simulink model "es2_Q2_task1"  (R2022b)
settings: Solver=VariableStepAuto  StartTime=0.0  StopTime=100.0  RelTol=1e-3  AbsTol=1e-3  EnableMultiTasking=on
undefined symbols (not defined in the file): X, Y, Z
libraries: nesl_utility x37, sm_lib x25
settings Model: Creator=matteo  LastModifiedBy=veronicagavagna
settings SolverCC: AutoScaleAbsTol=off  AlgebraicLoopSolver=TrustRegion  MaxZcPerStep=1
settings DataIOCC: LimitDataPoints=on  MaxDataPoints=10000
settings OptimizationCC: LifeSpan=inf
settings DebuggingCC: UnconnectedInputMsg=warning  UnconnectedOutputMsg=warning  UnconnectedLineMsg=warning  AllowSymbolicDim=off  SFUnexpectedBacktrackingDiag=warning  SFNoUnconditionalDefaultTransitionDiag=warning  SFExecutionAtInitializationDiag=none  ArithmeticOperatorsInVariantConditions=warning
settings ModelReferenceCC: EnableRefExpFcnMdlSchedulingChecks=on
settings SFSimCC: SimUseLocalCustomCode=off  CustomCodeUndefinedFunction=UseInterfaceOnly
settings RTWCC: RTWUseLocalCustomCode=off  DLArmComputeVersion=19.05
settings CodeAppCC: StateflowObjectComments=on
settings GRTTargetCC: TargetLangStandard=C89/C90 (ANSI)
settings ConfigComp: CovMetricSettings=dw  CovSaveCumulativeToWorkspaceVar=on  CovSaveSingleToWorkspaceVar=on  CovExternalEMLEnable=off  CovSFcnEnable=off
settings SimscapeCC: SimscapeLogType=all  SimscapeLogSimulationStatistics=on  SimscapeLogDataHistory=10000

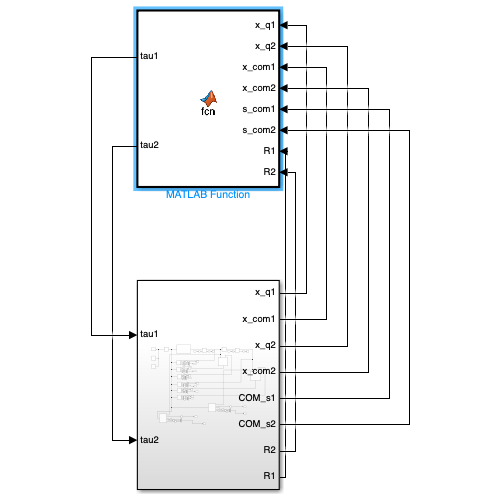
[thumbnail: Simulink's stored preview of the top-level diagram]
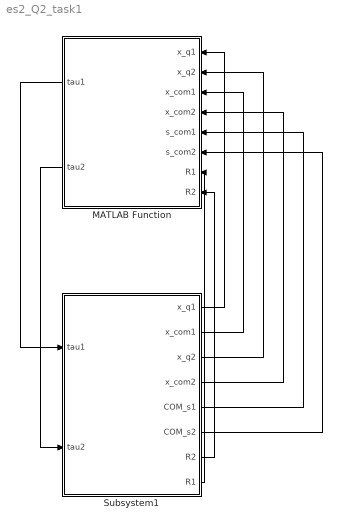
== system es2_Q2_task1 ==
  MATLAB Function : MATLAB Function  TreatAsAtomicUnit=on
  Subsystem1 : Subsystem
  wires:
  Subsystem1/1(x_q1) -> MATLAB Function/1(x_q1)
  Subsystem1/2(x_com1) -> MATLAB Function/3(x_com1)
  Subsystem1/3(x_q2) -> MATLAB Function/2(x_q2)
  Subsystem1/4(x_com2) -> MATLAB Function/4(x_com2)
  MATLAB Function/1(tau1) -> Subsystem1/1(tau1)
  MATLAB Function/2(tau2) -> Subsystem1/2(tau2)
  Subsystem1/5(COM_s1) -> MATLAB Function/5(s_com1)
  Subsystem1/6(COM_s2) -> MATLAB Function/6(s_com2)
  Subsystem1/7(R2) -> MATLAB Function/8(R2)
  Subsystem1/8(R1) -> MATLAB Function/7(R1)

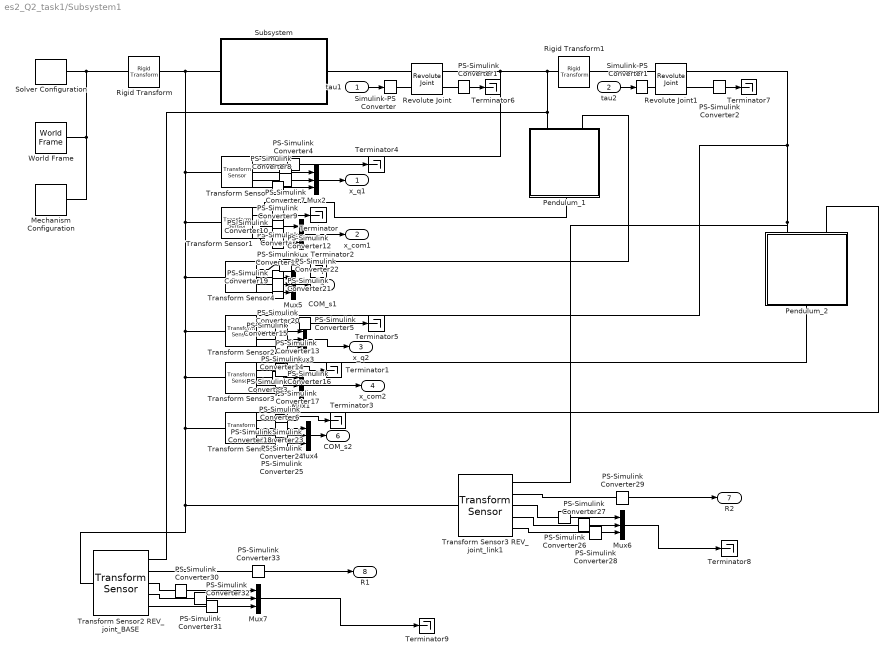
== system es2_Q2_task1/Subsystem1 ==
  tau1 : Inport
  tau2 : Inport  Port=2
  Mechanism Configuration : sm_lib/Utilities/Mechanism Configuration  UniformGravity=Constant  GravityVector=[0 0 -9.81]  GravityUnits=m/s^2  LinearizationDelta=0.001  JointModeTransitionNonlinearIterations=2
  Mux{,1..7} (8 alike) : Mux  Inputs=3
  PS-Simulink Converter{,1..33} (34 alike) : nesl_utility/PS-Simulink Converter  PhysicalDomain=network_engine_domain  SubClassName=ps_output  LeftPortType=input  RightPortType=output  PseudoPeriodic=off  Frequencies=[]  VectorFormat=inherit  Unit=inherit  AffineConversion=off
  Pendulum_1 : Subsystem
  Pendulum_2 : Subsystem
  Revolute Joint : sm_lib/Joints/Revolute Joint  JointMode=Normal  SenseConstraintForce=off  SenseConstraintForceX=off  SenseConstraintForceY=off  SenseConstraintForceZ=off  SenseConstraintTorque=off  SenseConstraintTorqueX=off  SenseConstraintTorqueY=off  SenseConstraintTorqueZ=off  SenseTotalForce=off  SenseTotalForceX=off  SenseTotalForceY=off  SenseTotalForceZ=off  SenseTotalTorque=off  SenseTotalTorqueX=off  SenseTotalTorqueY=off  SenseTotalTorqueZ=off  CompositeWrenchDir=FollowerOnBase  CompositeWrenchFrame=BaseFrame  EquilibriumPosition=0  EquilibriumPositionUnits=deg  SpringStiffness=0  SpringStiffnessUnits=N*m/deg  DampingCoefficient=0.002  DampingCoefficientUnits=N*m/(deg/s)  TorqueActuationMode=InputTorque  MotionActuationMode=ComputedMotion  SensePosition=on  SenseVelocity=off  SenseAcceleration=off  SenseTorqueForce=off  SenseLowerLimitTorqueForce=off  SenseUpperLimitTorqueForce=off  LowerLimitSpecify=off  LowerLimitBound=-90  LowerLimitBoundUnits=deg  LowerLimitStiffness=1e4  LowerLimitStiffnessUnits=N*m/deg  LowerLimitDamping=10  LowerLimitDampingUnits=N*m/(deg/s)  LowerLimitTransitionRegionWidth=0.1  LowerLimitTransitionRegionWidthUnits=deg  UpperLimitSpecify=off  UpperLimitBound=90  UpperLimitBoundUnits=deg  UpperLimitStiffness=1e4  UpperLimitStiffnessUnits=N*m/deg  UpperLimitDamping=10  UpperLimitDampingUnits=N*m/(deg/s)  UpperLimitTransitionRegionWidth=0.1  UpperLimitTransitionRegionWidthUnits=deg  PositionTargetSpecify=on  PositionTargetPriority=High  PositionTargetValue=30  PositionTargetValueUnits=deg  VelocityTargetSpecify=off  VelocityTargetPriority=High  VelocityTargetValue=0  VelocityTargetValueUnits=deg/s
  Revolute Joint1 : sm_lib/Joints/Revolute Joint  JointMode=Normal  SenseConstraintForce=off  SenseConstraintForceX=off  SenseConstraintForceY=off  SenseConstraintForceZ=off  SenseConstraintTorque=off  SenseConstraintTorqueX=off  SenseConstraintTorqueY=off  SenseConstraintTorqueZ=off  SenseTotalForce=off  SenseTotalForceX=off  SenseTotalForceY=off  SenseTotalForceZ=off  SenseTotalTorque=off  SenseTotalTorqueX=off  SenseTotalTorqueY=off  SenseTotalTorqueZ=off  CompositeWrenchDir=FollowerOnBase  CompositeWrenchFrame=BaseFrame  EquilibriumPosition=0  EquilibriumPositionUnits=deg  SpringStiffness=0  SpringStiffnessUnits=N*m/deg  DampingCoefficient=0.002  DampingCoefficientUnits=N*m/(deg/s)  TorqueActuationMode=InputTorque  MotionActuationMode=ComputedMotion  SensePosition=on  SenseVelocity=off  SenseAcceleration=off  SenseTorqueForce=off  SenseLowerLimitTorqueForce=off  SenseUpperLimitTorqueForce=off  LowerLimitSpecify=off  LowerLimitBound=-90  LowerLimitBoundUnits=deg  LowerLimitStiffness=1e4  LowerLimitStiffnessUnits=N*m/deg  LowerLimitDamping=10  LowerLimitDampingUnits=N*m/(deg/s)  LowerLimitTransitionRegionWidth=0.1  LowerLimitTransitionRegionWidthUnits=deg  UpperLimitSpecify=off  UpperLimitBound=90  UpperLimitBoundUnits=deg  UpperLimitStiffness=1e4  UpperLimitStiffnessUnits=N*m/deg  UpperLimitDamping=10  UpperLimitDampingUnits=N*m/(deg/s)  UpperLimitTransitionRegionWidth=0.1  UpperLimitTransitionRegionWidthUnits=deg  PositionTargetSpecify=on  PositionTargetPriority=High  PositionTargetValue=-30  PositionTargetValueUnits=deg  VelocityTargetSpecify=off  VelocityTargetPriority=High  VelocityTargetValue=0  VelocityTargetValueUnits=deg/s
  Rigid Transform : sm_lib/Frames and Transforms/Rigid Transform  TranslationMethod=None  TranslationStandardOffset=0  TranslationLengthUnit=m  TranslationStandardAxis=+Z  TranslationCartesianOffset=[0 0 0]  TranslationROffset=0  TranslationROffsetUnits=m  TranslationZOffset=0  TranslationZOffsetUnits=m  TranslationThetaOffset=0  TranslationThetaOffsetUnits=deg  RotationMethod=AlignedAxes  RotationAngleUnits=deg  RotationStandardAxis=+Z  RotationAngle=0.0  RotationArbitraryAxis=[0 0 1]  FollAlignAxisA=+X  BaseAlignAxisA=+Y  FollAlignAxisB=+Z  BaseAlignAxisB=+Z  RotationSequenceAxes=FollowerAxes  RotationSequence=XYX  RotationSequenceAngles=[0 0 0]  RotationSequenceAnglesUnits=deg  RotationMatrix=[1 0 0; 0 1 0; 0 0 1]  Quaternion=[1 0 0 0]
  Rigid Transform1 : sm_lib/Frames and Transforms/Rigid Transform  TranslationMethod=StandardAxis  TranslationStandardOffset=50  TranslationLengthUnit=cm  TranslationStandardAxis=-X  TranslationCartesianOffset=[0 0 0]  TranslationROffset=0  TranslationROffsetUnits=m  TranslationZOffset=0  TranslationZOffsetUnits=m  TranslationThetaOffset=0  TranslationThetaOffsetUnits=deg  RotationMethod=AlignedAxes  RotationAngleUnits=deg  RotationStandardAxis=+Z  RotationAngle=0.0  RotationArbitraryAxis=[0 0 1]  FollAlignAxisA=-Z  BaseAlignAxisA=+X  FollAlignAxisB=+Y  BaseAlignAxisB=+Y  RotationSequenceAxes=FollowerAxes  RotationSequence=XYX  RotationSequenceAngles=[0 0 0]  RotationSequenceAnglesUnits=deg  RotationMatrix=[1 0 0; 0 1 0; 0 0 1]  Quaternion=[1 0 0 0]
  Simulink-PS Converter : nesl_utility/Simulink-PS Converter  PhysicalDomain=network_engine_domain  SubClassName=ps_input  LeftPortType=input  RightPortType=output  PseudoPeriodic=off  Frequencies=[]  NoiseDistribution=none  NoiseParameters=[]  Unit=1  AffineConversion=off  FilteringAndDerivatives=provide  SimscapeFilterOrder=1  InputFilterTimeConstant=0.001  UdotUserProvided=0
  Simulink-PS Converter1 : nesl_utility/Simulink-PS Converter  PhysicalDomain=network_engine_domain  SubClassName=ps_input  LeftPortType=input  RightPortType=output  PseudoPeriodic=off  Frequencies=[]  NoiseDistribution=none  NoiseParameters=[]  Unit=1  AffineConversion=off  FilteringAndDerivatives=provide  SimscapeFilterOrder=1  InputFilterTimeConstant=0.001  UdotUserProvided=0
  Solver Configuration : nesl_utility/Solver Configuration  PhysicalDomain=network_engine_domain  SubClassName=solver  LeftPortType=input  RightPortType=generic  Tones=[]  Harmonics=[]  SimulateNoise=off  Profile=off  UseLocalSampling=off  EnableSwitchedLinearOptims=on  FrequencyDomain=off  UseCCode=off  RelTol=0.001  AbsTol=1e-06  MinStep=1e-09  ToWorkspace=off  RevertToSquareIcSolve=off  NumHomotopyIterations=100  PhasorMode=off  PhasorModeNumHarmonics=1  ConsistencySolver=NEWTON_XTOL_AFTER_FTOL  IndexReductionMethod=DerivativeReplacement  DoDC=off  ResidualTolerance=1e-09  ConsistencyTolSource=GLOBAL  ConsistencyAbsTol=0.001  ConsistencyRelTol=0.001  ConsistencyTolFactor=0.001  UseLocalSolver=off  LocalSolverChoice=NE_BACKWARD_EULER_ADVANCER  ResolveIndetEquations=on  FunctionEvalNumThread=1  LocalSolverSampleTime=0.001  DoFixedCost=off  MaxNonlinIter=3  MaxModeIter=2  ComputeImpulses=off  ImpulseIterations=2  LinearAlgebra=Sparse  LinearAlgebraNumThread=0  EquationFormulation=NE_TIME_EF  DelaysMemoryBudget=1024  AutomaticFiltering=on  FilteringTimeConstant=0.001  PartitionStorageMethod=AS_NEEDED  PartitionMemoryBudget=1024  PartitionMethod=FAST
  Subsystem : Subsystem
  Terminator{,1..9} (10 alike) : Terminator
  Transform Sensor{,1..5} (6 alike) : sm_lib/Frames and Transforms/Transform Sensor  MeasurementFrame=Base  SenseAngle=off  SenseAxis=off  SenseQ=off  SenseR=on  SenseRotationSequence=off  RotationSequence=XYX  SenseOmegaX=off  SenseOmegaY=off  SenseOmegaZ=off  SenseQDot=off  SenseRDot=off  SenseAlphaX=off  SenseAlphaY=off  SenseAlphaZ=off  SenseQDDot=off  SenseRDDot=off  SenseX=on  SenseY=on  SenseZ=on  SenseRad=off  SenseAzim=off  SenseDist=off  SenseInc=off  SenseXDot=off  SenseYDot=off  SenseZDot=off  SenseRadDot=off  SenseAzimDot=off  SenseDistDot=off  SenseIncDot=off  SenseXDDot=off  SenseYDDot=off  SenseZDDot=off  SenseRadDDot=off  SenseAzimDDot=off  SenseDistDDot=off  SenseIncDDot=off
  Transform Sensor2 REV_joint_BASE : sm_lib/Frames and Transforms/Transform Sensor  MeasurementFrame=Base  SenseAngle=off  SenseAxis=off  SenseQ=off  SenseR=on  SenseRotationSequence=off  RotationSequence=XYX  SenseOmegaX=off  SenseOmegaY=off  SenseOmegaZ=off  SenseQDot=off  SenseRDot=off  SenseAlphaX=off  SenseAlphaY=off  SenseAlphaZ=off  SenseQDDot=off  SenseRDDot=off  SenseX=on  SenseY=on  SenseZ=on  SenseRad=off  SenseAzim=off  SenseDist=off  SenseInc=off  SenseXDot=off  SenseYDot=off  SenseZDot=off  SenseRadDot=off  SenseAzimDot=off  SenseDistDot=off  SenseIncDot=off  SenseXDDot=off  SenseYDDot=off  SenseZDDot=off  SenseRadDDot=off  SenseAzimDDot=off  SenseDistDDot=off  SenseIncDDot=off
  Transform Sensor3 REV_joint_link1 : sm_lib/Frames and Transforms/Transform Sensor  MeasurementFrame=Base  SenseAngle=off  SenseAxis=off  SenseQ=off  SenseR=on  SenseRotationSequence=off  RotationSequence=XYX  SenseOmegaX=off  SenseOmegaY=off  SenseOmegaZ=off  SenseQDot=off  SenseRDot=off  SenseAlphaX=off  SenseAlphaY=off  SenseAlphaZ=off  SenseQDDot=off  SenseRDDot=off  SenseX=on  SenseY=on  SenseZ=on  SenseRad=off  SenseAzim=off  SenseDist=off  SenseInc=off  SenseXDot=off  SenseYDot=off  SenseZDot=off  SenseRadDot=off  SenseAzimDot=off  SenseDistDot=off  SenseIncDot=off  SenseXDDot=off  SenseYDDot=off  SenseZDDot=off  SenseRadDDot=off  SenseAzimDDot=off  SenseDistDDot=off  SenseIncDDot=off
  World Frame : sm_lib/Frames and Transforms/World Frame
  x_q1 : Outport
  x_com1 : Outport  Port=2
  x_q2 : Outport  Port=3
  x_com2 : Outport  Port=4
  COM_s1 : Outport  Port=5
  COM_s2 : Outport  Port=6
  R2 : Outport  Port=7
  R1 : Outport  Port=8
  wires:
  tau1/1 -> Simulink-PS Converter/1
  PS-Simulink Converter10/1 -> Mux/1
  PS-Simulink Converter2/1 -> Terminator7/1
  tau2/1 -> Simulink-PS Converter1/1
  PS-Simulink Converter5/1 -> Terminator5/1
  PS-Simulink Converter17/1 -> Mux1/2
  PS-Simulink Converter16/1 -> Mux1/1
  Mux1/1 -> x_com2/1
  PS-Simulink Converter1/1 -> Terminator6/1
  PS-Simulink Converter3/1 -> Terminator1/1
  PS-Simulink Converter15/1 -> Mux3/3
  PS-Simulink Converter8/1 -> Mux2/2
  PS-Simulink Converter11/1 -> Mux/2
  PS-Simulink Converter6/1 -> Mux1/3
  PS-Simulink Converter/1 -> Terminator/1
  PS-Simulink Converter12/1 -> Mux/3
  Mux/1 -> x_com1/1
  Mux3/1 -> x_q2/1
  PS-Simulink Converter4/1 -> Terminator4/1
  PS-Simulink Converter9/1 -> Mux2/3
  PS-Simulink Converter13/1 -> Mux3/1
  Mux2/1 -> x_q1/1
  PS-Simulink Converter7/1 -> Mux2/1
  PS-Simulink Converter14/1 -> Mux3/2
  PS-Simulink Converter19/1 -> Mux5/1
  PS-Simulink Converter21/1 -> Mux5/2
  PS-Simulink Converter20/1 -> Mux5/3
  PS-Simulink Converter22/1 -> Terminator2/1
  PS-Simulink Converter24/1 -> Mux4/1
  PS-Simulink Converter18/1 -> Mux4/2
  PS-Simulink Converter25/1 -> Mux4/3
  PS-Simulink Converter23/1 -> Terminator3/1
  Mux4/1 -> COM_s2/1
  Mux5/1 -> COM_s1/1
  PS-Simulink Converter26/1 -> Mux6/1
  Mux6/1 -> Terminator8/1
  PS-Simulink Converter29/1 -> R2/1
  PS-Simulink Converter27/1 -> Mux6/2
  PS-Simulink Converter28/1 -> Mux6/3
  PS-Simulink Converter33/1 -> R1/1
  PS-Simulink Converter30/1 -> Mux7/1
  PS-Simulink Converter31/1 -> Mux7/2
  PS-Simulink Converter32/1 -> Mux7/3
  Mux7/1 -> Terminator9/1
  connections:
  Transform Sensor1/RConn1 -- Pendulum_1/RConn1
  Transform Sensor/RConn3 -- PS-Simulink Converter7/LConn1
  Transform Sensor/RConn5 -- PS-Simulink Converter9/LConn1
  Transform Sensor1/RConn4 -- PS-Simulink Converter11/LConn1
  PS-Simulink Converter16/LConn1 -- Transform Sensor3/RConn3
  World Frame/RConn1 -- Rigid Transform/LConn1 -- Solver Configuration/RConn1 -- Mechanism Configuration/RConn1
  Transform Sensor2/RConn4 -- PS-Simulink Converter14/LConn1
  Subsystem/RConn1 -- Revolute Joint/LConn1
  Transform Sensor/RConn4 -- PS-Simulink Converter8/LConn1
  Revolute Joint1/RConn1 -- Transform Sensor2/RConn1 -- Transform Sensor3 REV_joint_link1/RConn1 -- Pendulum_2/LConn1
  Rigid Transform/RConn1 -- Subsystem/LConn1 -- Transform Sensor/LConn1 -- Transform Sensor1/LConn1 -- Transform Sensor4/LConn1 -- Transform Sensor2/LConn1 -- Transform Sensor3/LConn1 -- Transform Sensor2 REV_joint_BASE/LConn1 -- Transform Sensor3 REV_joint_link1/LConn1 -- Transform Sensor5/LConn1
  Transform Sensor1/RConn5 -- PS-Simulink Converter12/LConn1
  Revolute Joint/RConn2 -- PS-Simulink Converter1/LConn1
  Transform Sensor2/RConn5 -- PS-Simulink Converter15/LConn1
  Transform Sensor3/RConn2 -- PS-Simulink Converter3/LConn1
  Revolute Joint1/LConn1 -- Rigid Transform1/RConn1
  PS-Simulink Converter5/LConn1 -- Transform Sensor2/RConn2
  Revolute Joint1/RConn2 -- PS-Simulink Converter2/LConn1
  Simulink-PS Converter/RConn1 -- Revolute Joint/LConn2
  Transform Sensor3/RConn4 -- PS-Simulink Converter17/LConn1
  Simulink-PS Converter1/RConn1 -- Revolute Joint1/LConn2
  Transform Sensor3/RConn5 -- PS-Simulink Converter6/LConn1
  Transform Sensor2/RConn3 -- PS-Simulink Converter13/LConn1
  PS-Simulink Converter/LConn1 -- Transform Sensor1/RConn2
  Transform Sensor3/RConn1 -- Pendulum_2/RConn1
  PS-Simulink Converter10/LConn1 -- Transform Sensor1/RConn3
  PS-Simulink Converter4/LConn1 -- Transform Sensor/RConn2
  Transform Sensor4/RConn1 -- Pendulum_1/LConn2
  Transform Sensor5/RConn1 -- Pendulum_2/LConn2
  Transform Sensor4/RConn5 -- PS-Simulink Converter20/LConn1
  Transform Sensor4/RConn4 -- PS-Simulink Converter21/LConn1
  Transform Sensor4/RConn3 -- PS-Simulink Converter19/LConn1
  Transform Sensor4/RConn2 -- PS-Simulink Converter22/LConn1
  Transform Sensor5/RConn2 -- PS-Simulink Converter23/LConn1
  Transform Sensor5/RConn3 -- PS-Simulink Converter24/LConn1
  Transform Sensor5/RConn4 -- PS-Simulink Converter18/LConn1
  Transform Sensor5/RConn5 -- PS-Simulink Converter25/LConn1
  Revolute Joint/RConn1 -- Rigid Transform1/LConn1 -- Transform Sensor2 REV_joint_BASE/RConn1 -- Pendulum_1/LConn1 -- Transform Sensor/RConn1
  Transform Sensor3 REV_joint_link1/RConn2 -- PS-Simulink Converter29/LConn1
  Transform Sensor3 REV_joint_link1/RConn5 -- PS-Simulink Converter28/LConn1
  Transform Sensor3 REV_joint_link1/RConn4 -- PS-Simulink Converter27/LConn1
  Transform Sensor3 REV_joint_link1/RConn3 -- PS-Simulink Converter26/LConn1
  Transform Sensor2 REV_joint_BASE/RConn3 -- PS-Simulink Converter30/LConn1
  Transform Sensor2 REV_joint_BASE/RConn5 -- PS-Simulink Converter32/LConn1
  Transform Sensor2 REV_joint_BASE/RConn2 -- PS-Simulink Converter33/LConn1
  Transform Sensor2 REV_joint_BASE/RConn4 -- PS-Simulink Converter31/LConn1

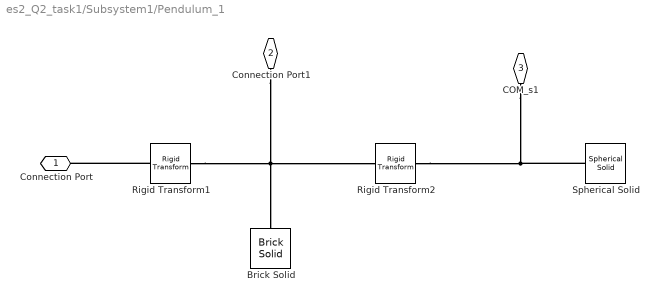
== system es2_Q2_task1/Subsystem1/Pendulum_1 ==
  Brick Solid : sm_lib/Body Elements/Brick Solid  GraphicAmbientColor=[0.15 0.15 0.15 1.0]  BasedOnType=Mass  BrickDimensions=[50 5 5]  BrickDimensionUnits=cm  CenterOfMass=[0 0 0]  CenterOfMassUnits=m  GraphicDiffuseColor=[0.5 0.5 0.5]  Density=1000  DensityUnits=kg/m^3  DoExposeReferenceFrame=on  GraphicEmissiveColor=[0.0 0.0 0.0 1.0]  ExportEntireGeometry=off  SerializedFrames=<Frames/>  MarkerShape=Sphere  MarkerSize=10  GraphicType=FromGeometry  InertiaType=CalculateFromGeometry  Mass=2  MassUnits=kg  MomentsOfInertia=[1 1 1]  MomentsOfInertiaUnits=kg*m^2  GraphicOpacity=1.0  ProductsOfInertia=[0 0 0]  ProductsOfInertiaUnits=kg*m^2  GraphicShininess=75  GraphicSpecularColor=[0.5 0.5 0.5 1.0]  GraphicVisPropType=SimpleVisualProperties
  Rigid Transform1 : sm_lib/Frames and Transforms/Rigid Transform  TranslationMethod=StandardAxis  TranslationStandardOffset=50/2  TranslationLengthUnit=cm  TranslationStandardAxis=+X  TranslationCartesianOffset=[0 0 0]  TranslationROffset=0  TranslationROffsetUnits=m  TranslationZOffset=0  TranslationZOffsetUnits=m  TranslationThetaOffset=0  TranslationThetaOffsetUnits=deg  RotationMethod=None  RotationAngleUnits=deg  RotationStandardAxis=+Z  RotationAngle=0.0  RotationArbitraryAxis=[0 0 1]  FollAlignAxisA=+Z  BaseAlignAxisA=+X  FollAlignAxisB=+Y  BaseAlignAxisB=+Y  RotationSequenceAxes=FollowerAxes  RotationSequence=XYX  RotationSequenceAngles=[0 0 0]  RotationSequenceAnglesUnits=deg  RotationMatrix=[1 0 0; 0 1 0; 0 0 1]  Quaternion=[1 0 0 0]
  Rigid Transform2 : sm_lib/Frames and Transforms/Rigid Transform  TranslationMethod=StandardAxis  TranslationStandardOffset=50/2  TranslationLengthUnit=cm  TranslationStandardAxis=-X  TranslationCartesianOffset=[0 0 0]  TranslationROffset=0  TranslationROffsetUnits=m  TranslationZOffset=0  TranslationZOffsetUnits=m  TranslationThetaOffset=0  TranslationThetaOffsetUnits=deg  RotationMethod=AlignedAxes  RotationAngleUnits=deg  RotationStandardAxis=+Z  RotationAngle=0.0  RotationArbitraryAxis=[0 0 1]  FollAlignAxisA=-Z  BaseAlignAxisA=+X  FollAlignAxisB=+Y  BaseAlignAxisB=+Y  RotationSequenceAxes=FollowerAxes  RotationSequence=XYX  RotationSequenceAngles=[0 0 0]  RotationSequenceAnglesUnits=deg  RotationMatrix=[1 0 0; 0 1 0; 0 0 1]  Quaternion=[1 0 0 0]
  Spherical Solid : sm_lib/Body Elements/Spherical Solid  GraphicAmbientColor=[0.15 0.15 0.15 1.0]  BasedOnType=Mass  CenterOfMass=[0 0 0]  CenterOfMassUnits=m  GraphicDiffuseColor=[0.5 0.5 0.5]  Density=10000  DensityUnits=kg/m^3  DoExposeReferenceFrame=on  GraphicEmissiveColor=[0.0 0.0 0.0 1.0]  ExportEntireGeometry=off  SerializedExposedGeometries=<ExposedGeometries/>  SerializedFrames=<Frames/>  MarkerShape=Sphere  MarkerSize=10  GraphicType=FromGeometry  InertiaType=CalculateFromGeometry  Mass=0  MassUnits=kg  MomentsOfInertia=[1 1 1]  MomentsOfInertiaUnits=kg*m^2  GraphicOpacity=1.0  ProductsOfInertia=[0 0 0]  ProductsOfInertiaUnits=kg*m^2  GraphicShininess=75  GraphicSpecularColor=[0.5 0.5 0.5 1.0]  SphereRadius=5  SphereRadiusUnits=cm  GraphicVisPropType=SimpleVisualProperties
  Connection Port : PMIOPort  Side=Left
  Connection Port1 : PMIOPort  Port=2  Side=Right
  COM_s1 : PMIOPort  Port=3  Side=Left
  connections:
  Rigid Transform2/RConn1 -- Spherical Solid/RConn1 -- COM_s1/RConn1
  Rigid Transform1/LConn1 -- Connection Port1/RConn1 -- Rigid Transform2/LConn1 -- Brick Solid/RConn1
  Rigid Transform1/RConn1 -- Connection Port/RConn1

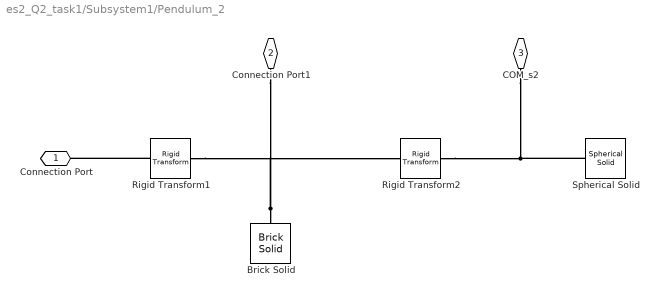
== system es2_Q2_task1/Subsystem1/Pendulum_2 ==
  Brick Solid : sm_lib/Body Elements/Brick Solid  GraphicAmbientColor=[0.15 0.15 0.15 1.0]  BasedOnType=Mass  BrickDimensions=[30 5 5]  BrickDimensionUnits=cm  CenterOfMass=[0 0 0]  CenterOfMassUnits=m  GraphicDiffuseColor=[0.5 0.5 0.5]  Density=1000  DensityUnits=kg/m^3  DoExposeReferenceFrame=on  GraphicEmissiveColor=[0.0 0.0 0.0 1.0]  ExportEntireGeometry=off  SerializedFrames=<Frames/>  MarkerShape=Sphere  MarkerSize=10  GraphicType=FromGeometry  InertiaType=CalculateFromGeometry  Mass=1  MassUnits=kg  MomentsOfInertia=[1 1 1]  MomentsOfInertiaUnits=kg*m^2  GraphicOpacity=1.0  ProductsOfInertia=[0 0 0]  ProductsOfInertiaUnits=kg*m^2  GraphicShininess=75  GraphicSpecularColor=[0.5 0.5 0.5 1.0]  GraphicVisPropType=SimpleVisualProperties
  Rigid Transform1 : sm_lib/Frames and Transforms/Rigid Transform  TranslationMethod=StandardAxis  TranslationStandardOffset=30/2  TranslationLengthUnit=cm  TranslationStandardAxis=+X  TranslationCartesianOffset=[0 0 0]  TranslationROffset=0  TranslationROffsetUnits=m  TranslationZOffset=0  TranslationZOffsetUnits=m  TranslationThetaOffset=0  TranslationThetaOffsetUnits=deg  RotationMethod=None  RotationAngleUnits=deg  RotationStandardAxis=+Z  RotationAngle=0.0  RotationArbitraryAxis=[0 0 1]  FollAlignAxisA=+Z  BaseAlignAxisA=+X  FollAlignAxisB=+Y  BaseAlignAxisB=+Y  RotationSequenceAxes=FollowerAxes  RotationSequence=XYX  RotationSequenceAngles=[0 0 0]  RotationSequenceAnglesUnits=deg  RotationMatrix=[1 0 0; 0 1 0; 0 0 1]  Quaternion=[1 0 0 0]
  Rigid Transform2 : sm_lib/Frames and Transforms/Rigid Transform  TranslationMethod=StandardAxis  TranslationStandardOffset=30/2  TranslationLengthUnit=cm  TranslationStandardAxis=-X  TranslationCartesianOffset=[0 0 0]  TranslationROffset=0  TranslationROffsetUnits=m  TranslationZOffset=0  TranslationZOffsetUnits=m  TranslationThetaOffset=0  TranslationThetaOffsetUnits=deg  RotationMethod=None  RotationAngleUnits=deg  RotationStandardAxis=+Z  RotationAngle=0.0  RotationArbitraryAxis=[0 0 1]  FollAlignAxisA=+X  BaseAlignAxisA=+Y  FollAlignAxisB=+Y  BaseAlignAxisB=+Z  RotationSequenceAxes=FollowerAxes  RotationSequence=XYX  RotationSequenceAngles=[0 0 0]  RotationSequenceAnglesUnits=deg  RotationMatrix=[1 0 0; 0 1 0; 0 0 1]  Quaternion=[1 0 0 0]
  Spherical Solid : sm_lib/Body Elements/Spherical Solid  GraphicAmbientColor=[0.15 0.15 0.15 1.0]  BasedOnType=Mass  CenterOfMass=[0 0 0]  CenterOfMassUnits=m  GraphicDiffuseColor=[0.5 0.5 0.5]  Density=10000  DensityUnits=kg/m^3  DoExposeReferenceFrame=on  GraphicEmissiveColor=[0.0 0.0 0.0 1.0]  ExportEntireGeometry=off  SerializedExposedGeometries=<ExposedGeometries/>  SerializedFrames=<Frames/>  MarkerShape=Sphere  MarkerSize=10  GraphicType=FromGeometry  InertiaType=CalculateFromGeometry  Mass=2  MassUnits=kg  MomentsOfInertia=[1 1 1]  MomentsOfInertiaUnits=kg*m^2  GraphicOpacity=1.0  ProductsOfInertia=[0 0 0]  ProductsOfInertiaUnits=kg*m^2  GraphicShininess=75  GraphicSpecularColor=[0.5 0.5 0.5 1.0]  SphereRadius=5  SphereRadiusUnits=cm  GraphicVisPropType=SimpleVisualProperties
  Connection Port : PMIOPort  Side=Left
  Connection Port1 : PMIOPort  Port=2  Side=Right
  COM_s2 : PMIOPort  Port=3  Side=Left
  connections:
  COM_s2/RConn1 -- Spherical Solid/RConn1 -- Rigid Transform2/RConn1
  Brick Solid/RConn1 -- Connection Port1/RConn1 -- Rigid Transform1/LConn1 -- Rigid Transform2/LConn1
  Rigid Transform1/RConn1 -- Connection Port/RConn1

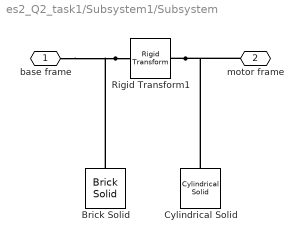
== system es2_Q2_task1/Subsystem1/Subsystem ==
  Brick Solid : sm_lib/Body Elements/Brick Solid  GraphicAmbientColor=[0.15 0.15 0.15 1.0]  BasedOnType=Density  BrickDimensions=[30 30 10]  BrickDimensionUnits=cm  CenterOfMass=[0 0 0]  CenterOfMassUnits=m  GraphicDiffuseColor=[0.5 0.5 0.5]  Density=1000  DensityUnits=kg/m^3  DoExposeReferenceFrame=on  GraphicEmissiveColor=[0.0 0.0 0.0 1.0]  ExportEntireGeometry=off  SerializedFrames=<Frames/>  MarkerShape=Sphere  MarkerSize=10  GraphicType=FromGeometry  InertiaType=CalculateFromGeometry  Mass=1  MassUnits=kg  MomentsOfInertia=[1 1 1]  MomentsOfInertiaUnits=kg*m^2  GraphicOpacity=1.0  ProductsOfInertia=[0 0 0]  ProductsOfInertiaUnits=kg*m^2  GraphicShininess=75  GraphicSpecularColor=[0.5 0.5 0.5 1.0]  GraphicVisPropType=SimpleVisualProperties
  Cylindrical Solid : sm_lib/Body Elements/Cylindrical Solid  GraphicAmbientColor=[0.15 0.15 0.15 1.0]  BasedOnType=Density  CenterOfMass=[0 0 0]  CenterOfMassUnits=m  GraphicDiffuseColor=[0.5 0.5 0.5]  CylinderLength=10  CylinderLengthUnits=cm  CylinderRadius=5  CylinderRadiusUnits=cm  Density=1000  DensityUnits=kg/m^3  DoExposeReferenceFrame=on  GraphicEmissiveColor=[0.0 0.0 0.0 1.0]  ExportEntireGeometry=off  SerializedFrames=<Frames/>  MarkerShape=Sphere  MarkerSize=10  GraphicType=FromGeometry  InertiaType=CalculateFromGeometry  Mass=1  MassUnits=kg  MomentsOfInertia=[1 1 1]  MomentsOfInertiaUnits=kg*m^2  GraphicOpacity=1.0  ProductsOfInertia=[0 0 0]  ProductsOfInertiaUnits=kg*m^2  GraphicShininess=75  GraphicSpecularColor=[0.5 0.5 0.5 1.0]  GraphicVisPropType=SimpleVisualProperties
  Rigid Transform1 : sm_lib/Frames and Transforms/Rigid Transform  TranslationMethod=StandardAxis  TranslationStandardOffset=10  TranslationLengthUnit=cm  TranslationStandardAxis=+Z  TranslationCartesianOffset=[0 0 0]  TranslationROffset=0  TranslationROffsetUnits=m  TranslationZOffset=0  TranslationZOffsetUnits=m  TranslationThetaOffset=0  TranslationThetaOffsetUnits=deg  RotationMethod=None  RotationAngleUnits=deg  RotationStandardAxis=+Z  RotationAngle=0.0  RotationArbitraryAxis=[0 0 1]  FollAlignAxisA=+Z  BaseAlignAxisA=-Y  FollAlignAxisB=+X  BaseAlignAxisB=+X  RotationSequenceAxes=FollowerAxes  RotationSequence=XYX  RotationSequenceAngles=[0 0 0]  RotationSequenceAnglesUnits=deg  RotationMatrix=[1 0 0; 0 1 0; 0 0 1]  Quaternion=[1 0 0 0]
  base frame : PMIOPort  Side=Left
  motor frame : PMIOPort  Port=2  Side=Right
  connections:
  Rigid Transform1/RConn1 -- motor frame/RConn1 -- Cylindrical Solid/RConn1
  Rigid Transform1/LConn1 -- base frame/RConn1 -- Brick Solid/RConn1

== matlab function es2_Q2_task1/MATLAB Function ==
  data: tau1 output; x_q1 input; x_q2 input; x_com1 input; x_com2 input; tau2 output; s_com1 input; s_com2 input; R1 input; R2 input
function [tau1,tau2]= fcn(x_q1,x_q2,x_com1,x_com2,s_com1,s_com2, R1, R2)

m1 = 2; %mass of the links1
m2 = 0; %mass of the sfera1
m3 = 1; %mass of the links2
m4 = 2; %mass of the sfera2

g1 = [0; 0; -9.81];

F1 = m1 * g1;
F2 = m2 * g1;
F3 = m3 * g1;
F4 = m4 * g1;
F = [F1; F2; F3; F4];

k1 = [0; 0; 1]; %along z

r_1_1_l = x_com1 - x_q1; %distanza asta1 e frame1
r_1_1_s = s_com1 - x_q1; %distanza sfera1 e frame 1
r_2_1_l = x_com2 - x_q1; %distanza asta2 e frame 1
r_2_1_s = s_com2 - x_q1; %distanza sfera2 e frame1
r_2_2_l = x_com2 - x_q2; %distanza asta2 frame 2
r_2_2_s = s_com2 - x_q2; %distanza sfera2 e frame 2

J_l1 = [cross(R1*k1, r_1_1_l) zeros(3,1)]; %jacobiana asta1
J_l2 = [cross(R1*k1, r_1_1_s) zeros(3,1)]; %jacobiana sfera1
J_l3 = [cross(R1*k1, r_2_1_l) cross(R2*k1, r_2_2_l)]; %jacobiana asta2
J_l4 = [cross(R1*k1, r_2_1_s) cross(R2*k1, r_2_2_s)]; %jacoabiana sfera2


J = [J_l1', J_l2', J_l3', J_l4'];

tau = -J * F;

tau1 = tau(1,1);
tau2 = tau(2,1);
